simulink model "car_suspension"  (R2020a)
settings: Solver=ode45  StartTime=0.0  StopTime=5  RelTol=1e-3
values from neighbouring files (symbols this model uses):
  b = 1250    [car_suspension.m]    (also in main.m = 12500)
  K1 = 7500    [car_suspension.m]    (also in main.m)
  K2 = 170000    [car_suspension.m]    (also in main.m)
  M = 500    [car_suspension.m]    (also in main.m = 700)
settings Model: Creator=ACER  LastModifiedBy=ACER

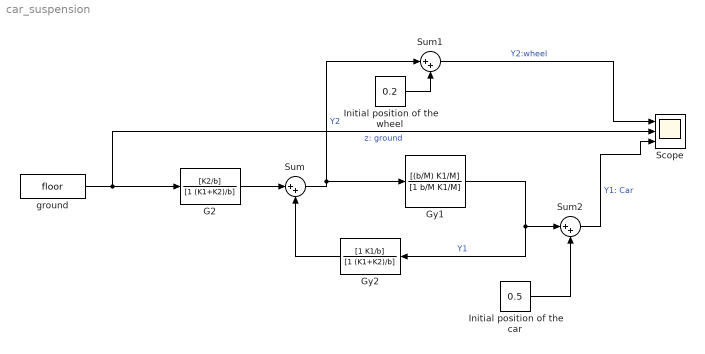
== system car_suspension ==
  G2 : TransferFcn  Numerator=[K2/b]  Denominator=[1 (K1+K2)/b]
  Gy1 : TransferFcn  Numerator=[(b/M) K1/M]  Denominator=[1 b/M K1/M]
  Gy2 : TransferFcn  Numerator=[1 K1/b]  Denominator=[1 (K1+K2)/b]
  Initial position of the car : Constant  Value=0.5
  Initial position of the wheel : Constant  Value=0.2
  Scope : Scope  NumInputPorts=3
  Sum : Sum  Inputs=|++
  Sum1 : Sum  Inputs=|++
  Sum2 : Sum  Inputs=|++
  ground : FromWorkspace  VariableName=floor
  wires:
  G2/1 -> Sum/1
  Sum/1 -> Sum1/1, Gy1/1  "Y2"
  Gy1/1 -> Sum2/1, Gy2/1  "Y1"
  Gy2/1 -> Sum/2
  ground/1 -> Scope/2, G2/1  "z: ground"
  Sum1/1 -> Scope/1  "Y2:wheel"
  Initial position of the car/1 -> Sum2/2
  Sum2/1 -> Scope/3  "Y1: Car"
  Initial position of the wheel/1 -> Sum1/2
